simulink model "mcb_microchip_pmsm_parameter_est_host_SAME70"  (R2023b)
settings: Solver=FixedStepDiscrete  StartTime=0.0  StopTime=inf  RelTol=1e-3  EnableMultiTasking=on
values from neighbouring files (symbols this model uses):
  Ts = T_pwm    (= 5e-05)    [mcb_microchip_pmsm_parameter_est_SAME70_data.m]
  Ts_SerialCom = 0.0005    [mcb_microchip_pmsm_parameter_est_SAME70_data.m]
undefined symbols (not defined in the file or in its folder): pmsm, target
libraries: simulink x4, instrumentseriallib x3, mcbpmsmparamestlib x1, svdutilitieslib x1
settings Model: Creator=The MathWorks, Inc.  LastModifiedBy=I69995
settings SolverCC: AlgebraicLoopSolver=TrustRegion
settings DataIOCC: LimitDataPoints=on  SaveFormat=Array  ReturnWorkspaceOutputs=off
settings OptimizationCC: LifeSpan=1  EfficientTunableParamExpr=on
settings DebuggingCC: MergeDetectMultiDrivingBlocksExec=none  SolverPrmCheckMsg=warning  ParameterPrecisionLossMsg=none  UnconnectedInputMsg=warning  UnconnectedOutputMsg=warning  UnconnectedLineMsg=warning  AllowSymbolicDim=off  PregeneratedLibrarySubsystemCodeDiagnostic=none  SFUnexpectedBacktrackingDiag=warning  SFNoUnconditionalDefaultTransitionDiag=warning  SFExecutionAtInitializationDiag=none  ArithmeticOperatorsInVariantConditions=warning
settings HardwareCC: ProdBitPerPointer=32  ProdLargestAtomicFloat=None  ProdIntDivRoundTo=Undefined  ProdEndianess=Unspecified  ProdWordSize=32  ProdHWDeviceType=32-bit Generic
settings ModelReferenceCC: EnableRefExpFcnMdlSchedulingChecks=on  PropagateSignalLabelsOutOfModel=off
settings SFSimCC: SimUseLocalCustomCode=off  MATLABDynamicMemAlloc=off
settings RTWCC: Description=Real-Time Workshop Embedded Coder  SystemTargetFile=ert.tlc  TemplateMakefile=ert_default_tmf  GenerateReport=on  RTWUseLocalCustomCode=off  IncludeHyperlinkInReport=on  LaunchReport=on  GenerateTraceInfo=on  GenerateTraceReport=on  GenerateTraceReportSl=on  GenerateTraceReportSf=on  GenerateTraceReportEml=on  DLArmComputeVersion=19.05
settings CodeAppCC: IgnoreCustomStorageClasses=off  StateflowObjectComments=on  InternalIdentifier=Classic
settings ERTTargetCC: MultiwordLength=2048  GenerateSampleERTMain=on  ERTCustomFileTemplate=example_file_process.tlc  ConvertIfToSwitch=off  SuppressUnreachableDefaultCases=off
settings ConfigComp: CovMetricSettings=dw  CovSaveCumulativeToWorkspaceVar=on  CovSaveSingleToWorkspaceVar=on  CovExternalEMLEnable=off  CovSFcnEnable=off

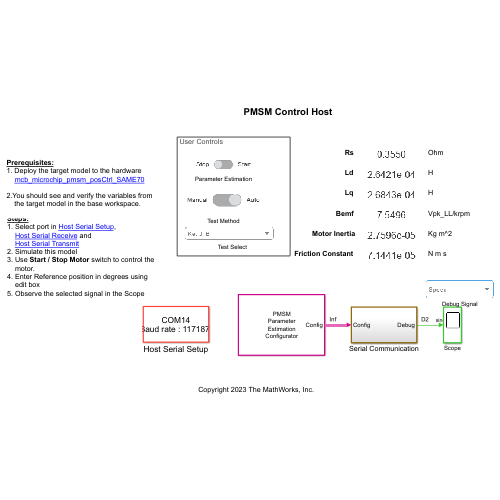
[thumbnail: Simulink's stored preview of the top-level diagram]
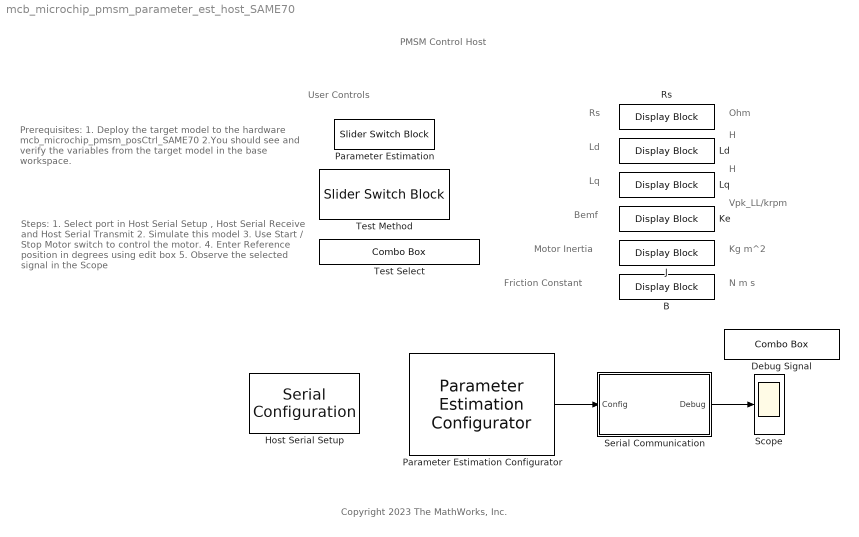
== system mcb_microchip_pmsm_parameter_est_host_SAME70 ==
  note: PMSM Control Host
  note: Copyright 2023 The MathWorks, Inc.
  note: Prerequisites:
      | 1. Deploy the target model to the hardware
      | mcb_microchip_pmsm_posCtrl_SAME70
      |
      | 2.You should see and verify the variables from
      | the target model in the base workspace.
  note: Steps:
      | 1. Select port in Host Serial Setup ,
      | Host Serial Receive and
      | Host Serial Transmit
      | 2. Simulate this model
      | 3. Use Start / Stop Motor switch to control the
      | motor.
      | 4. Enter Reference position in degrees using
      | edit box
      | 5. Observe the selected signal in the Scope
  note: User Controls
  note: Lq
  note: H
  note: H
  note: Ohm
  note: Motor Inertia
  note: N m s
  note: Rs
  note: Friction Constant
  note: Vpk_LL/krpm
  note: Bemf
  note: Ld
  note: Kg m^2
  B : DisplayBlock  LabelPosition=Hide  Transparency=1
  Debug Signal : ComboBox  LabelPosition=Hide  SelectedLabel=Speed
      settings: Values={{'Speed', 'Ia', 'Ib', 'Theta', 'Ld_PhaseDiff_deg', 'Lq_PhaseDiff_deg', 'Vd_RsTest', 'Id_LdTest', 'Vd_LdTest', 'InjFreq_LdTest', 'PhaseDiff_LdTest', 'Iq_LqTest', 'Vq_LqTest', 'InjFreq_LqTest', 'PhaseDiff_LqTest', 'Vd', 'Vq', 'Id', 'Iq', 'CoastDown Time'}, [1 2 3 4 5 6 7 8 9 10 11 12 13 14 15 16 17 18 19 20]}
  Host Serial Setup : instrumentseriallib/Serial Configuration  Priority=-99  PortSel=COM14  Port=COM14  ComPort=COM14  BaudRate=1171875  DataBits=8  Parity=none  StopBits=1  ByteOrder=little-endian  FlowControl=none  Timeout=2  SimulateUsing=Interpreted execution  BlockInModel=on  aMode=5
  J : DisplayBlock  LabelPosition=Hide  Transparency=1
  Ke : DisplayBlock  LabelPosition=Hide  Transparency=1
  Ld : DisplayBlock  LabelPosition=Hide  Transparency=1
  Lq : DisplayBlock  LabelPosition=Hide  Transparency=1
  Parameter Estimation : SliderSwitchBlock  LabelPosition=Hide
      settings: Values={{'Stop', 'Start'}, [0 1]}
  Parameter Estimation Configurator : mcbpmsmparamestlib/Parameter Estimation Configurator  P=pmsm.p  NRated=pmsm.N_rated  IRated=pmsm.I_rated  ImaxInverter=inverter.ISenseMax  RBoard=inverter.R_board  ISenseGain=inverter.AmpPerCount  VSenseGain=inverter.VoltPerCount  FreqMax=1000  FreqMin=400  FreqStepSweep=100  FreqStepEst=10  FreqNum=10  KeTime=5  KeSpeed=0.9 * pmsm.N_rated  IqRefFOC=0.2  KpKiInputEnable=off  Kp=1  Ki=10  JSpeedLow=0.2 * pmsm.N_rated  DataType=single  Ts=Ts
      settings: LibrarySourceBlock=mcblib/Parameter Estimation/PMSM Parameter Estimation/Parameter Estimation Configurator
  Rs : DisplayBlock  LabelPosition=Hide  Transparency=1
  Scope : Scope
  Serial Communication : Subsystem
  Test Method : SliderSwitchBlock  LabelPosition=Hide
      settings: Values={{'Manual', 'Auto'}, [0 1]}
  Test Select : ComboBox  LabelPosition=Hide  SelectedLabel=Ke, J, B
      settings: Values={{'No Test', 'Rs', 'Ld', 'Lq', 'Ke, J, B'}, [0 1 2 3 4]}
  wires:
  Serial Communication/1(Debug) -> Scope/1
  Parameter Estimation Configurator/1 -> Serial Communication/1(Config)

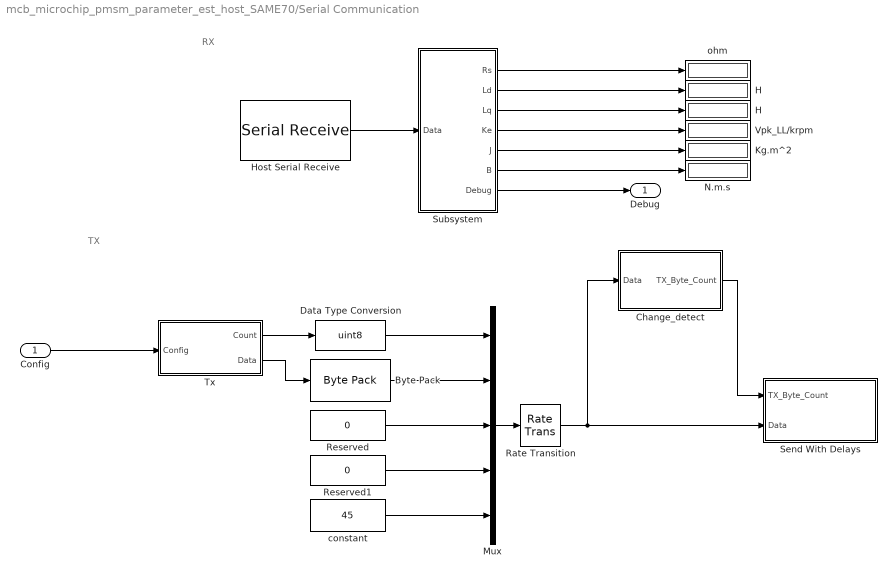
== system mcb_microchip_pmsm_parameter_est_host_SAME70/Serial Communication ==
  note: RX
  note: TX
  Config : Inport
  Byte Pack : svdutilitieslib/Byte Pack  maskPackedDataType=uint8  datatypes={'single'}  byteAlign=1  blockPlatform=tic2000
  Change_detect : Subsystem
  Data Type Conversion : DataTypeConversion  OutDataTypeStr=uint8  RndMeth=Simplest  SaturateOnIntegerOverflow=off
  H : Display
      settings: Format=short_e
  "H " : Display
      settings: Format=short_e
  Host Serial Receive : instrumentseriallib/Serial Receive  PortSel=COM14  Port=COM14  ComPort=COM14  DataType=single  SaveDataType=uint8  ToggleHeader=on  Header='ES'  ToggleTerminator=off  Terminator=<none>  CustomTerminator='E'  InputFormat=Row major  ToggleDataSize=on  DataSize=[target.SerialFrameSize 3]  EnableBlockingMode=on  ActionDataUnavailable=Output custom value  ActionWhenDataUnavailable=Output custom value  CustomValue=15  SampleTime=Ts_SerialCom * target.SerialFrameSize  SimulateUsing=Interpreted execution  BlockInModel=on  aMode=5
  Kg.m^2 : Display
      settings: Format=short_e
  Mux : Mux  Inputs=5
  N.m.s : Display
      settings: Format=short_e
  Rate Transition : RateTransition  OutPortSampleTime=0.002
  Reserved : Constant  Value=0  VectorParams1D=off  OutDataTypeStr=uint8  SampleTime=Ts_SerialCom * target.SerialFrameSize
  Reserved1 : Constant  Value=0  VectorParams1D=off  OutDataTypeStr=uint8  SampleTime=Ts_SerialCom * target.SerialFrameSize
  Send With Delays : Subsystem
  Subsystem : Subsystem
  Tx : Subsystem
  Vpk_LL/krpm : Display
      settings: Format=short_e
  constant : Constant  Value=45  VectorParams1D=off  OutDataTypeStr=uint8  SampleTime=Ts_SerialCom * target.SerialFrameSize
  ohm : Display
      settings: Format=short_e
  Debug : Outport
  wires:
  Host Serial Receive/1 -> Subsystem/1(Data)
  Change_detect/1(TX_Byte_Count) -> Send With Delays/1(TX_Byte_Count)
  Subsystem/1(Rs) -> ohm/1
  Subsystem/2(Ld) -> H/1
  Subsystem/3(Lq) -> "H "/1
  Subsystem/4(Ke) -> Vpk_LL/krpm/1
  Subsystem/5(J) -> Kg.m^2/1
  Subsystem/6(B) -> N.m.s/1
  Tx/1(Count) -> Data Type Conversion/1
  Tx/2(Data) -> Byte Pack/1
  Subsystem/7(Debug) -> Debug/1
  Reserved/1 -> Mux/3
  Reserved1/1 -> Mux/4
  constant/1 -> Mux/5
  Byte Pack/1 -> Mux/2
  Data Type Conversion/1 -> Mux/1
  Mux/1 -> Rate Transition/1
  Rate Transition/1 -> Change_detect/1(Data), Send With Delays/2(Data)
  Config/1 -> Tx/1(Config)

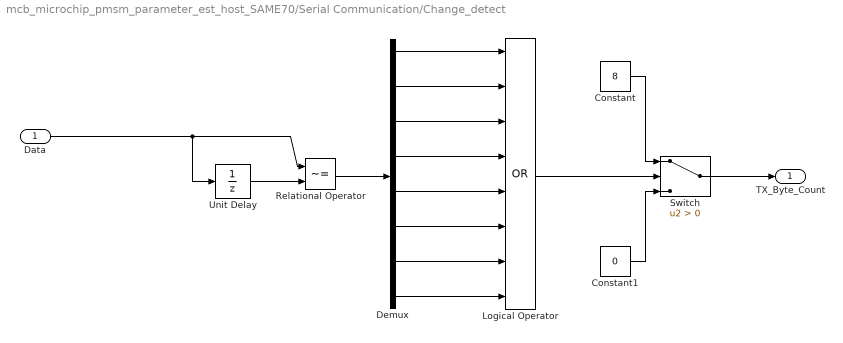
== system mcb_microchip_pmsm_parameter_est_host_SAME70/Serial Communication/Change_detect ==
  Data : Inport
  Constant : Constant  Value=8  OutDataTypeStr=uint8
  Constant1 : Constant  Value=0  OutDataTypeStr=uint8
  Demux : Demux  Outputs=8
  Logical Operator : Logic  Operator=OR  Inputs=8  AllPortsSameDT=off  OutDataTypeStr=boolean
  Relational Operator : RelationalOperator  Operator=~=  OutDataTypeStr=boolean  InputSameDT=off
  Switch : Switch  Criteria=u2 > Threshold  SaturateOnIntegerOverflow=off  InputSameDT=off
  Unit Delay : UnitDelay  InitialCondition=0.5  SampleTime=-1  HasFrameUpgradeWarning=on
  TX_Byte_Count : Outport  VectorParamsAs1DForOutWhenUnconnected=off
  wires:
  Data/1 -> Relational Operator/1, Unit Delay/1
  Unit Delay/1 -> Relational Operator/2
  Constant1/1 -> Switch/3
  Constant/1 -> Switch/1
  Relational Operator/1 -> Demux/1
  Switch/1 -> TX_Byte_Count/1
  Demux/1 -> Logical Operator/1
  Demux/2 -> Logical Operator/2
  Demux/4 -> Logical Operator/4
  Demux/3 -> Logical Operator/3
  Demux/5 -> Logical Operator/5
  Demux/6 -> Logical Operator/6
  Demux/7 -> Logical Operator/7
  Demux/8 -> Logical Operator/8
  Logical Operator/1 -> Switch/2

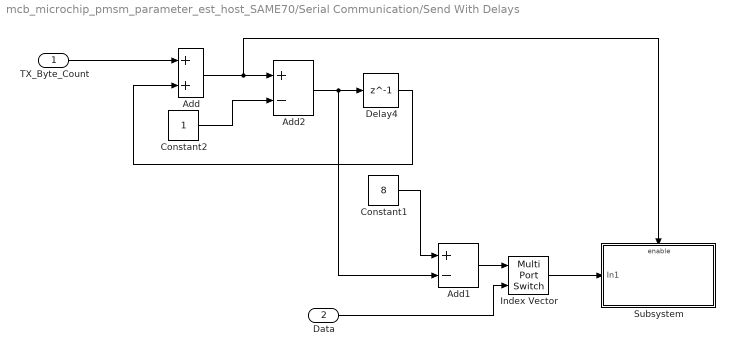
== system mcb_microchip_pmsm_parameter_est_host_SAME70/Serial Communication/Send With Delays ==
  TX_Byte_Count : Inport
  Data : Inport  Port=2
  Add : Sum  SaturateOnIntegerOverflow=on
  Add1 : Sum  Inputs=+-  SaturateOnIntegerOverflow=on
  Add2 : Sum  Inputs=+-  SaturateOnIntegerOverflow=on
  Constant1 : Constant  Value=8  OutDataTypeStr=uint8
  Constant2 : Constant  OutDataTypeStr=uint8
  Delay4 : Delay  DelayLength=1
  Index Vector : MultiPortSwitch  Inputs=1  SaturateOnIntegerOverflow=off  InputSameDT=off
  Subsystem : Subsystem
  wires:
  Data/1 -> Index Vector/2
  TX_Byte_Count/1 -> Add/1
  Add/1 -> Subsystem/Enable, Add2/1
  Delay4/1 -> Add/2
  Add1/1 -> Index Vector/1
  Constant1/1 -> Add1/1
  Index Vector/1 -> Subsystem/1(In1)
  Add2/1 -> Add1/2, Delay4/1
  Constant2/1 -> Add2/2

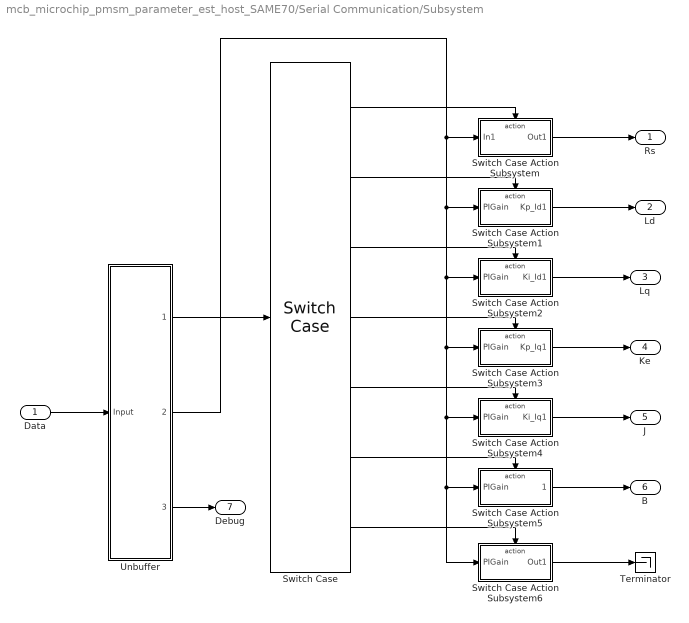
== system mcb_microchip_pmsm_parameter_est_host_SAME70/Serial Communication/Subsystem ==
  Data : Inport
  Switch Case : SwitchCase  CaseConditions={1, 2, 3, 4, 5, 6}
  Switch Case Action Subsystem : Subsystem  TreatAsAtomicUnit=on
  Switch Case Action Subsystem1 : Subsystem  TreatAsAtomicUnit=on
  Switch Case Action Subsystem2 : Subsystem  TreatAsAtomicUnit=on
  Switch Case Action Subsystem3 : Subsystem  TreatAsAtomicUnit=on
  Switch Case Action Subsystem4 : Subsystem  TreatAsAtomicUnit=on
  Switch Case Action Subsystem5 : Subsystem  TreatAsAtomicUnit=on
  Switch Case Action Subsystem6 : Subsystem  TreatAsAtomicUnit=on
  Terminator : Terminator
  Unbuffer : MATLAB Function  TreatAsAtomicUnit=on
  Rs : Outport
  Ld : Outport  Port=2
  Lq : Outport  Port=3
  Ke : Outport  Port=4
  J : Outport  Port=5
  B : Outport  Port=6
  Debug : Outport  Port=7
  wires:
  Switch Case/1 -> Switch Case Action Subsystem/Action
  Unbuffer/2(Output2) -> Switch Case Action Subsystem6/1(PIGain), Switch Case Action Subsystem5/1(PIGain), Switch Case Action Subsystem4/1(PIGain), Switch Case Action Subsystem3/1(PIGain), Switch Case Action Subsystem2/1(PIGain), Switch Case Action Subsystem1/1(PIGain), Switch Case Action Subsystem/1(In1)
  Switch Case/2 -> Switch Case Action Subsystem1/Action
  Switch Case/3 -> Switch Case Action Subsystem2/Action
  Switch Case/4 -> Switch Case Action Subsystem3/Action
  Switch Case/5 -> Switch Case Action Subsystem4/Action
  Switch Case/6 -> Switch Case Action Subsystem5/Action
  Switch Case/7 -> Switch Case Action Subsystem6/Action
  Switch Case Action Subsystem/1(Out1) -> Rs/1
  Switch Case Action Subsystem1/1(Kp_Id1) -> Ld/1
  Switch Case Action Subsystem2/1(Ki_Id1) -> Lq/1
  Switch Case Action Subsystem3/1(Kp_Iq1) -> Ke/1
  Switch Case Action Subsystem4/1(Ki_Iq1) -> J/1
  Switch Case Action Subsystem5/1(Kp_Speed1) -> B/1
  Switch Case Action Subsystem6/1(Out1) -> Terminator/1
  Data/1 -> Unbuffer/1(Input)
  Unbuffer/1(Output1) -> Switch Case/1
  Unbuffer/3(Output3) -> Debug/1

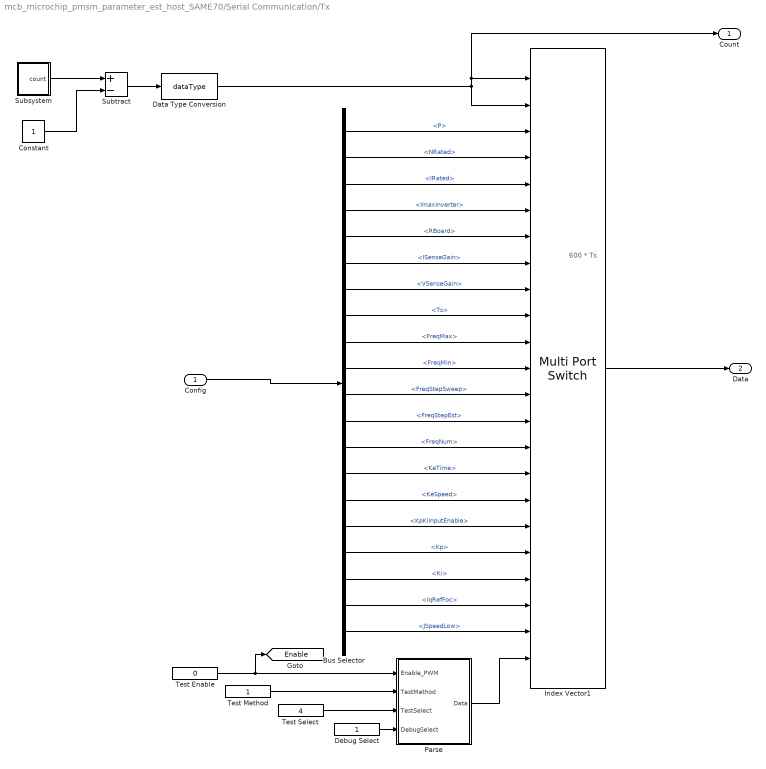
== system mcb_microchip_pmsm_parameter_est_host_SAME70/Serial Communication/Tx ==
  note: 600 * Ts
  Config : Inport
  Bus Selector : BusSelector  OutputSignals=P,NRated,IRated,ImaxInverter,RBoard,ISenseGain,VSenseGain,Ts,FreqMax,FreqMin,FreqStepSweep,FreqStepEst,FreqNum,KeTime,KeSpeed,KpKiInputEnable,Kp,Ki,IqRefFoc,JSpeedLow
  Constant : Constant  SampleTime=Ts_SerialCom * target.SerialFrameSize
  Data Type Conversion : DataTypeConversion  OutDataTypeStr=dataType  RndMeth=Simplest  SaturateOnIntegerOverflow=off
  Debug Select : Constant  OutDataTypeStr=uint16  SampleTime=Ts_SerialCom * target.SerialFrameSize
  Index Vector1 : MultiPortSwitch  DataPortOrder=Zero-based contiguous  Inputs=22  zeroidx=on  OutDataTypeStr=dataType  RndMeth=Simplest  SaturateOnIntegerOverflow=off  InputSameDT=off
  Parse : Subsystem
  Subsystem : Subsystem  mask(Counter){upperLimit=22, sampleTime=Ts_SerialCom * target.SerialFrameSize}
      mask prompts: upperLimit "Upper Limit"; sampleTime "Sample Time"
      mask help: Conter starts from 1 and reaches Upper Limit using given sample time in steps of 1.
  Subtract : Sum  Inputs=+-
  Test Enable : Constant  Value=0  VectorParams1D=off  OutDataTypeStr=uint16  SampleTime=Ts_SerialCom * target.SerialFrameSize
  Test Method : Constant  VectorParams1D=off  OutDataTypeStr=uint16  SampleTime=Ts_SerialCom * target.SerialFrameSize
  Test Select : Constant  Value=4  OutDataTypeStr=uint16  SampleTime=Ts_SerialCom * target.SerialFrameSize
  Count : Outport
  Data : Outport  Port=2
  tag scope: Enable=global
  wires:
  Config/1 -> Bus Selector/1
  Test Select/1 -> Parse/3(TestSelect)
  Test Method/1 -> Parse/2(TestMethod)
  Subsystem/1(count) -> Subtract/1
  Index Vector1/1 -> Data/1
  Data Type Conversion/1 -> Index Vector1/2, Count/1, Index Vector1/1
  Bus Selector/2 -> Index Vector1/4  "<NRated>"
  Bus Selector/1 -> Index Vector1/3  "<P>"
  Bus Selector/3 -> Index Vector1/5  "<IRated>"
  Bus Selector/4 -> Index Vector1/6  "<ImaxInverter>"
  Bus Selector/5 -> Index Vector1/7  "<RBoard>"
  Bus Selector/6 -> Index Vector1/8  "<ISenseGain>"
  Bus Selector/7 -> Index Vector1/9  "<VSenseGain>"
  Bus Selector/8 -> Index Vector1/10  "<Ts>"
  Bus Selector/9 -> Index Vector1/11  "<FreqMax>"
  Bus Selector/10 -> Index Vector1/12  "<FreqMin>"
  Debug Select/1 -> Parse/4(DebugSelect)
  Test Enable/1 -> [Enable], Parse/1(Enable_PWM)
  Parse/1(Data) -> Index Vector1/23
  Constant/1 -> Subtract/2
  Subtract/1 -> Data Type Conversion/1
  Bus Selector/11 -> Index Vector1/13  "<FreqStepSweep>"
  Bus Selector/12 -> Index Vector1/14  "<FreqStepEst>"
  Bus Selector/13 -> Index Vector1/15  "<FreqNum>"
  Bus Selector/14 -> Index Vector1/16  "<KeTime>"
  Bus Selector/15 -> Index Vector1/17  "<KeSpeed>"
  Bus Selector/16 -> Index Vector1/18  "<KpKiInputEnable>"
  Bus Selector/17 -> Index Vector1/19  "<Kp>"
  Bus Selector/18 -> Index Vector1/20  "<Ki>"
  Bus Selector/19 -> Index Vector1/21  "<IqRefFoc>"
  Bus Selector/20 -> Index Vector1/22  "<JSpeedLow>"

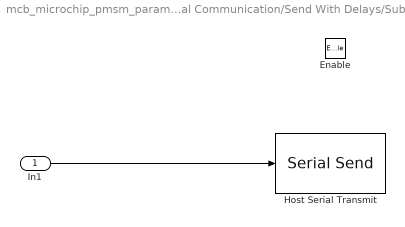
== system mcb_microchip_pmsm_parameter_est_host_SAME70/Serial Communication/Send With Delays/Subsystem ==
  In1 : Inport
  Enable : EnablePort
  Host Serial Transmit : instrumentseriallib/Serial Send  PortSel=COM14  Port=COM14  ComPort=COM14  Header=[]  Terminator=<none>  CustomTerminator=[]  EnableBlockingMode=off  SimulateUsing=Interpreted execution  BlockInModel=on  aMode=5
  wires:
  In1/1 -> Host Serial Transmit/1

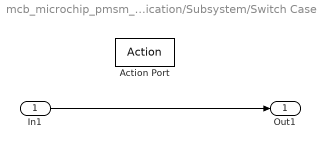
== system mcb_microchip_pmsm_parameter_est_host_SAME70/Serial Communication/Subsystem/Switch Case Action Subsystem ==
  In1 : Inport
  Action Port : ActionPort  ActionPortLabel=case [ 1 ]:
  Out1 : Outport
  wires:
  In1/1 -> Out1/1

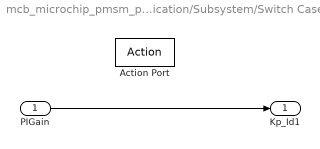
== system mcb_microchip_pmsm_parameter_est_host_SAME70/Serial Communication/Subsystem/Switch Case Action Subsystem1 ==
  PIGain : Inport
  Action Port : ActionPort  ActionPortLabel=case [ 2 ]:
  Kp_Id1 : Outport
  wires:
  PIGain/1 -> Kp_Id1/1

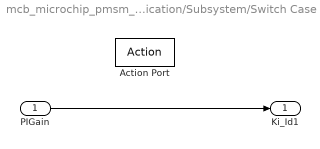
== system mcb_microchip_pmsm_parameter_est_host_SAME70/Serial Communication/Subsystem/Switch Case Action Subsystem2 ==
  PIGain : Inport
  Action Port : ActionPort  ActionPortLabel=case [ 3 ]:
  Ki_Id1 : Outport
  wires:
  PIGain/1 -> Ki_Id1/1

== system mcb_microchip_pmsm_parameter_est_host_SAME70/Serial Communication/Subsystem/Switch Case Action Subsystem3 ==
  PIGain : Inport
  Action Port : ActionPort  ActionPortLabel=case [ 4 ]:
  Kp_Iq1 : Outport
  wires:
  PIGain/1 -> Kp_Iq1/1

== system mcb_microchip_pmsm_parameter_est_host_SAME70/Serial Communication/Subsystem/Switch Case Action Subsystem4 ==
  PIGain : Inport
  Action Port : ActionPort  ActionPortLabel=case [ 5 ]:
  Ki_Iq1 : Outport
  wires:
  PIGain/1 -> Ki_Iq1/1

== system mcb_microchip_pmsm_parameter_est_host_SAME70/Serial Communication/Subsystem/Switch Case Action Subsystem5 ==
  PIGain : Inport
  Action Port : ActionPort  ActionPortLabel=case [ 6 ]:
  Kp_Speed1 : Outport
  wires:
  PIGain/1 -> Kp_Speed1/1

== system mcb_microchip_pmsm_parameter_est_host_SAME70/Serial Communication/Subsystem/Switch Case Action Subsystem6 ==
  PIGain : Inport
  Action Port : ActionPort  ActionPortLabel=default:
  Out1 : Outport
  wires:
  PIGain/1 -> Out1/1

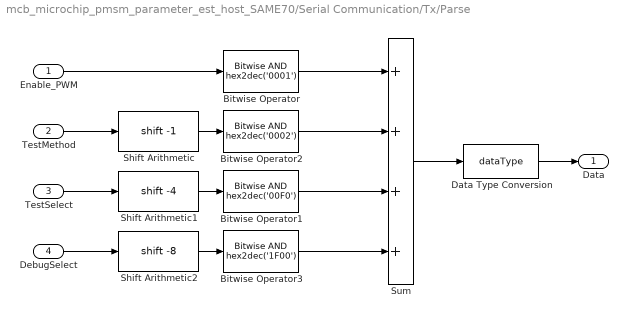
== system mcb_microchip_pmsm_parameter_est_host_SAME70/Serial Communication/Tx/Parse ==
  Enable_PWM : Inport
  TestMethod : Inport  Port=2
  TestSelect : Inport  Port=3
  DebugSelect : Inport  Port=4
  Bitwise Operator : simulink/Logic and Bit Operations/Bitwise Operator  logicop=AND  UseBitMask=on  BitMask=hex2dec('0001')  BitMaskRealWorld=Stored Integer
  Bitwise Operator1 : simulink/Logic and Bit Operations/Bitwise Operator  logicop=AND  UseBitMask=on  BitMask=hex2dec('00F0')  BitMaskRealWorld=Stored Integer
  Bitwise Operator2 : simulink/Logic and Bit Operations/Bitwise Operator  logicop=AND  UseBitMask=on  BitMask=hex2dec('0002')  BitMaskRealWorld=Stored Integer
  Bitwise Operator3 : simulink/Logic and Bit Operations/Bitwise Operator  logicop=AND  UseBitMask=on  BitMask=hex2dec('1F00')  BitMaskRealWorld=Stored Integer
  Data Type Conversion : DataTypeConversion  OutDataTypeStr=dataType  RndMeth=Simplest  SaturateOnIntegerOverflow=off
  Shift Arithmetic : ArithShift  BitShiftNumber=-1
  Shift Arithmetic1 : ArithShift  BitShiftNumber=-4
  Shift Arithmetic2 : ArithShift  BitShiftNumber=-8
  Sum : Sum  Inputs=++++
  Data : Outport
  wires:
  Bitwise Operator/1 -> Sum/1
  TestSelect/1 -> Shift Arithmetic1/1
  Sum/1 -> Data Type Conversion/1
  Shift Arithmetic1/1 -> Bitwise Operator1/1
  Shift Arithmetic/1 -> Bitwise Operator2/1
  Bitwise Operator1/1 -> Sum/3
  TestMethod/1 -> Shift Arithmetic/1
  Bitwise Operator2/1 -> Sum/2
  Enable_PWM/1 -> Bitwise Operator/1
  Data Type Conversion/1 -> Data/1
  DebugSelect/1 -> Shift Arithmetic2/1
  Shift Arithmetic2/1 -> Bitwise Operator3/1
  Bitwise Operator3/1 -> Sum/4

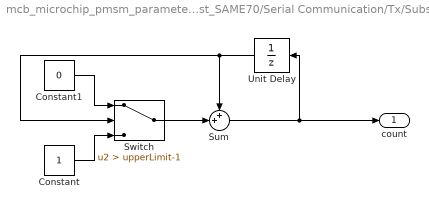
== system mcb_microchip_pmsm_parameter_est_host_SAME70/Serial Communication/Tx/Subsystem ==
  Constant : Constant  OutDataTypeStr=uint8  SampleTime=sampleTime
  Constant1 : Constant  Value=0  OutDataTypeStr=uint8  SampleTime=sampleTime
  Sum : Sum  Inputs=++|  OutDataTypeStr=uint8  AccumDataTypeStr=uint8  RndMeth=Simplest
  Switch : Switch  Criteria=u2 > Threshold  Threshold=upperLimit-1  OutDataTypeStr=uint8  RndMeth=Simplest  SaturateOnIntegerOverflow=off  InputSameDT=off
  Unit Delay : UnitDelay  SampleTime=-1  HasFrameUpgradeWarning=on
  count : Outport
  wires:
  Constant1/1 -> Switch/1
  Sum/1 -> count/1, Unit Delay/1
  Unit Delay/1 -> Switch/2, Sum/1
  Switch/1 -> Sum/2
  Constant/1 -> Switch/3

== matlab function mcb_microchip_pmsm_parameter_est_host_SAME70/Serial Communication/Subsystem/Unbuffer ==
  data: Input input; Output1 output; Output2 output; Output3 output
function [ Output1, Output2, Output3] = unBuf(Input)

selSignal = Input(:, 1);
Output1= selSignal(1,1);

selSignal = Input(:, 2);
Output2 = selSignal(1,1);

Output3 = Input(:, 3);

end
